simulink model "Question2"  (R2022b)
settings: Solver=ode4  StartTime=0.0  StopTime=tstop  FixedStep=tstep  RelTol=1e-3
undefined symbols (not defined in the file): C, L, R
settings Model: Creator=dipte  LastModifiedBy=dipte
settings DataIOCC: ReturnWorkspaceOutputs=off

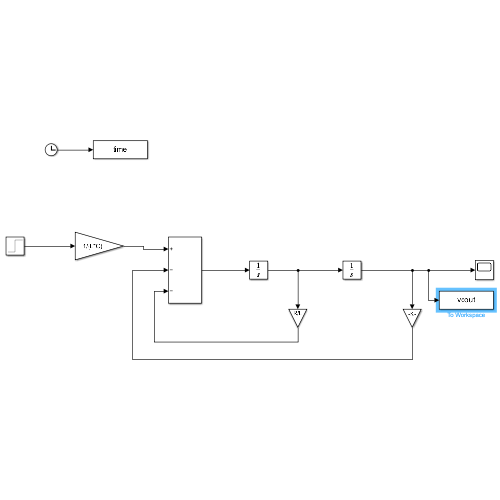
[thumbnail: Simulink's stored preview of the top-level diagram]
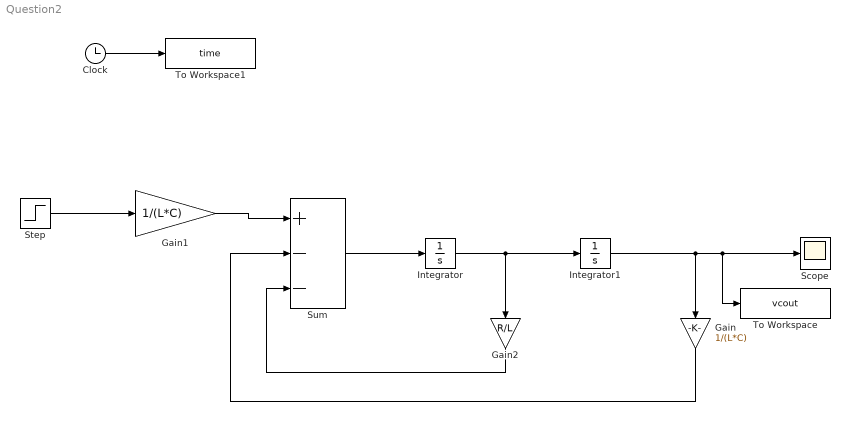
== system Question2 ==
  Clock : Clock
  Gain : Gain  Gain=1/(L*C)
  Gain1 : Gain  Gain=1/(L*C)
  Gain2 : Gain  Gain=R/L
  Integrator : Integrator
  Integrator1 : Integrator
  Scope : Scope
  Step : Step  Time=0  SampleTime=0
  Sum : Sum  Inputs=+--
  To Workspace : ToWorkspace  VariableName=vcout  SampleTime=-1
      settings: Save2DSignal=2-D array (concatenate along first dimension)
  To Workspace1 : ToWorkspace  VariableName=time  SampleTime=-1
      settings: Save2DSignal=2-D array (concatenate along first dimension)
  wires:
  Step/1 -> Gain1/1
  Gain1/1 -> Sum/1
  Sum/1 -> Integrator/1
  Integrator/1 -> Gain2/1, Integrator1/1
  Integrator1/1 -> Gain/1, To Workspace/1, Scope/1
  Gain2/1 -> Sum/3
  Gain/1 -> Sum/2
  Clock/1 -> To Workspace1/1
